simulink model "lab_2"  (R2016a)
settings: Solver=VariableStepAuto  SolverMode=SingleTasking  StartTime=0.0  StopTime=50  RelTol=1e-3
settings Model: Creator=Универская хуета  LastModifiedBy=Универская хуета
settings DataIOCC: LimitDataPoints=on  SaveOutput=off  SaveTime=off
settings OptimizationCC: BlockReduction=off  BooleanDataType=off
settings DebuggingCC: SaveWithParameterizedLinksMsg=none  UnderspecifiedInitializationDetection=Classic  MergeDetectMultiDrivingBlocksExec=none  SignalResolutionControl=TryResolveAllWithWarning  AllowSymbolicDim=off
settings HardwareCC: TargetBitPerPointer=64  TargetLongLongMode=on  TargetIntDivRoundTo=Zero  TargetEndianess=LittleEndian  TargetWordSize=64  TargetHWDeviceType=MATLAB Host  ProdEqTarget=off

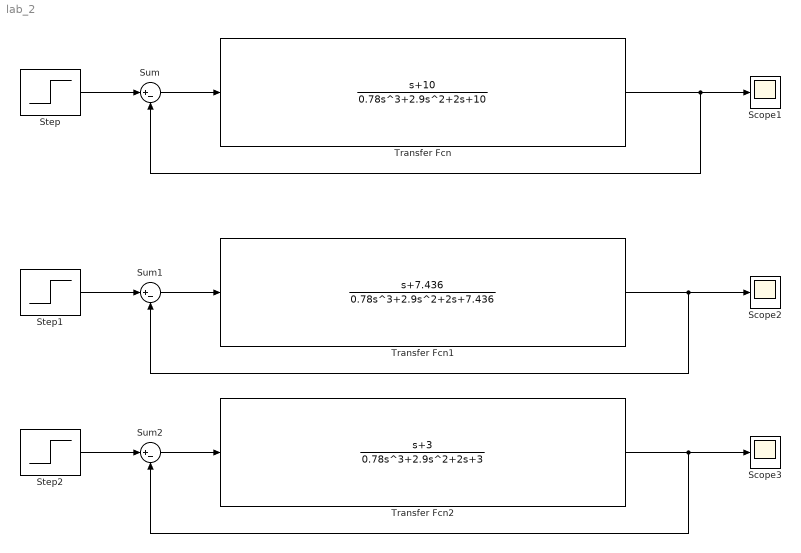
== system lab_2 ==
  Scope1 : Scope
  Scope2 : Scope
  Scope3 : Scope
  Step : Step  SampleTime=0
  Step1 : Step  SampleTime=0
  Step2 : Step  SampleTime=0
  Sum : Sum  Inputs=|+-
  Sum1 : Sum  Inputs=|+-
  Sum2 : Sum  Inputs=|+-
  Transfer Fcn : TransferFcn  Numerator=[1 10]  Denominator=[0.78 2.9 2 10]
  Transfer Fcn1 : TransferFcn  Numerator=[1 7.436]  Denominator=[0.78 2.9 2 7.436]
  Transfer Fcn2 : TransferFcn  Numerator=[1 3]  Denominator=[0.78 2.9 2 3]
  wires:
  Step/1 -> Sum/1
  Transfer Fcn/1 -> Sum/2, Scope1/1
  Step1/1 -> Sum1/1
  Transfer Fcn1/1 -> Scope2/1, Sum1/2
  Step2/1 -> Sum2/1
  Transfer Fcn2/1 -> Scope3/1, Sum2/2
  Sum/1 -> Transfer Fcn/1
  Sum1/1 -> Transfer Fcn1/1
  Sum2/1 -> Transfer Fcn2/1
